simulink model "InertiaWheelSystem2"  (R2014a)
settings: Solver=ode45  StartTime=0.0  StopTime=10.0  RelTol=1e-3
undefined symbols (not defined in the file or in its folder): Kt, N, Tdt, Tit
libraries: simulink x1, cstblocks x1
settings Model: Creator=elt11jke  LastModifiedBy=computerMaster_92
settings DataIOCC: SignalLoggingSaveFormat=ModelDataLogs
settings OptimizationCC: ExpressionDepthLimit=2147483647
settings DebuggingCC: UnderspecifiedInitializationDetection=Classic  FcnCallInpInsideContextMsg=EnableAllAsWarning  StateNameClashWarn=warning

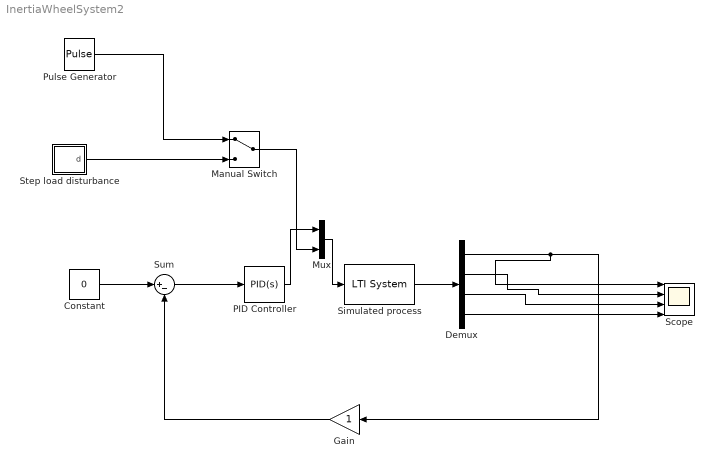
== system InertiaWheelSystem2 ==
  Constant : Constant  Value=0
  Demux : Demux
  Gain : Gain
  Manual Switch : ManualSwitch
  Mux : Mux  Inputs=2
  PID Controller : simulink/Continuous/PID Controller  Controller=PID  TimeDomain=Continuous-time  SampleTime=1  IntegratorMethod=Forward Euler  FilterMethod=Forward Euler  Form=Parallel  P=Kt  I=Tit  D=Tdt  N=N  InitialConditionSource=internal  InitialConditionForIntegrator=0  InitialConditionForFilter=0  ExternalReset=none  LimitOutput=off  UpperSaturationLimit=inf  LowerSaturationLimit=-inf  LinearizeAsGain=off  AntiWindupMode=none  Kb=1  TrackingMode=off  Kt=1  PParamMin=[]  PParamMax=[]  IParamMin=[]  IParamMax=[]  DParamMin=[]  DParamMax=[]  NParamMin=[]  NParamMax=[]  KbParamMin=[]  KbParamMax=[]  KtParamMin=[]  KtParamMax=[]  POutMin=[]  POutMax=[]  IOutMin=[]  IOutMax=[]  DOutMin=[]  DOutMax=[]  NOutMin=[]  NOutMax=[]  KbOutMin=[]  KbOutMax=[]  KtOutMin=[]  KtOutMax=[]  IntegratorOutMin=[]  IntegratorOutMax=[]  FilterOutMin=[]  FilterOutMax=[]  SumOutMin=[]  SumOutMax=[]  SumI1OutMin=[]  SumI1OutMax=[]  SumI2OutMin=[]  SumI2OutMax=[]  SumI3OutMin=[]  SumI3OutMax=[]  SumDOutMin=[]  SumDOutMax=[]  SaturationOutMin=[]  SaturationOutMax=[]  IntegratorContinuousStateAttributes=''  IntegratorStateMustResolveToSignalObject=off  IntegratorRTWStateStorageClass=Auto  FilterContinuousStateAttributes=''  FilterStateMustResolveToSignalObject=off  FilterRTWStateStorageClass=Auto
  Pulse Generator : DiscretePulseGenerator  PulseType=Time based  Amplitude=0.01  PulseWidth=5
  Scope : Scope  NumInputPorts=4
      settings: YMin=-5~-5~-5~-5  YMax=5~5~5~5
  Simulated process : cstblocks/LTI System  sys=Pin  IC=[]
  Step load disturbance : Subsystem
  Sum : Sum  Inputs=|+-
  wires:
  Sum/1 -> PID Controller/1
  Gain/1 -> Sum/2
  Step load disturbance/1(d) -> Manual Switch/2
  Pulse Generator/1 -> Manual Switch/1
  Constant/1 -> Sum/1
  Simulated process/1 -> Demux/1
  Demux/1 -> Gain/1, Scope/1
  Demux/3 -> Scope/3
  Demux/2 -> Scope/2
  Demux/4 -> Scope/4
  Manual Switch/1 -> Mux/2
  PID Controller/1 -> Mux/1
  Mux/1 -> Simulated process/1

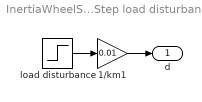
== system InertiaWheelSystem2/Step load disturbance ==
  1/km1 : Gain  Gain=0.01  SaturateOnIntegerOverflow=on  OutDataTypeStr=Inherit: Same as input  ParamDataTypeStr=Inherit: Same as input
  load disturbance : Step  Time=5  After=-0.15  SampleTime=0
  d : Outport
  wires:
  load disturbance/1 -> 1/km1/1
  1/km1/1 -> d/1
